simulink library "halin"  (R2021b)
settings: Solver=VariableStepAuto  StartTime=0.0  StopTime=10.0  RelTol=1e-3
undefined symbols (not defined in the file): TRUE
libraries: FVT_lib x177, hcu_lib x55
(part 13 of 17)

== system halin/HAL_IN/CAN1/ESC1/RFPulseCount ==
  RF_PulseCount : Inport
  UnitConverter : DataTypeConversion  OutDataTypeStr=uint8
  VHAL_RFPulseCount_enum : Outport
  wires:
  UnitConverter/1 -> VHAL_RFPulseCount_enum/1
  RF_PulseCount/1 -> UnitConverter/1

== system halin/HAL_IN/CAN1/ESC1/RFPulseCountV ==
  RF_PulseCount_V : Inport
  UnitConverter : DataTypeConversion  OutDataTypeStr=uint8
  VHAL_RFPulseCountV_flg : Outport
  wires:
  UnitConverter/1 -> VHAL_RFPulseCountV_flg/1
  RF_PulseCount_V/1 -> UnitConverter/1

== system halin/HAL_IN/CAN1/ESC1/RFRawWhlSpeed ==
  RF_RawWhlSpeed : Inport
  UnitConverter : DataTypeConversion  OutDataTypeStr=uint16
  convert_in : FVT_lib/hal/convert_in  gain=0.0625  offset=0
  VHAL_RFRawWhlSpeed_kph : Outport
  wires:
  convert_in/1 -> VHAL_RFRawWhlSpeed_kph/1
  UnitConverter/1 -> convert_in/1
  RF_RawWhlSpeed/1 -> UnitConverter/1

== system halin/HAL_IN/CAN1/ESC1/RFRawWhlSpeedV ==
  RF_RawWhlSpeed_V : Inport
  UnitConverter : DataTypeConversion  OutDataTypeStr=uint8
  VHAL_RFRawWhlSpeedV_flg : Outport
  wires:
  UnitConverter/1 -> VHAL_RFRawWhlSpeedV_flg/1
  RF_RawWhlSpeed_V/1 -> UnitConverter/1

== system halin/HAL_IN/CAN1/ESC1/RFWhlRotDir ==
  RF_WhlRotDir : Inport
  UnitConverter : DataTypeConversion  OutDataTypeStr=uint8
  VHAL_RFWhlRotDir_enum : Outport
  wires:
  UnitConverter/1 -> VHAL_RFWhlRotDir_enum/1
  RF_WhlRotDir/1 -> UnitConverter/1

== system halin/HAL_IN/CAN1/ESC1/RRPulseCount ==
  RR_PulseCount : Inport
  UnitConverter : DataTypeConversion  OutDataTypeStr=uint8
  VHAL_RRPulseCount_enum : Outport
  wires:
  UnitConverter/1 -> VHAL_RRPulseCount_enum/1
  RR_PulseCount/1 -> UnitConverter/1

== system halin/HAL_IN/CAN1/ESC1/RRPulseCountV ==
  RR_PulseCount_V : Inport
  UnitConverter : DataTypeConversion  OutDataTypeStr=uint8
  VHAL_RRPulseCountV_flg : Outport
  wires:
  UnitConverter/1 -> VHAL_RRPulseCountV_flg/1
  RR_PulseCount_V/1 -> UnitConverter/1

== system halin/HAL_IN/CAN1/ESC1/RRRawWhlSpeed ==
  RR_RawWhlSpeed : Inport
  UnitConverter : DataTypeConversion  OutDataTypeStr=uint16
  convert_in : FVT_lib/hal/convert_in  gain=0.0625  offset=0
  VHAL_RRRawWhlSpeed_kph : Outport
  wires:
  convert_in/1 -> VHAL_RRRawWhlSpeed_kph/1
  UnitConverter/1 -> convert_in/1
  RR_RawWhlSpeed/1 -> UnitConverter/1

== system halin/HAL_IN/CAN1/ESC1/RRRawWhlSpeedV ==
  RR_RawWhlSpeed_V : Inport
  UnitConverter : DataTypeConversion  OutDataTypeStr=uint8
  VHAL_RRRawWhlSpeedV_flg : Outport
  wires:
  UnitConverter/1 -> VHAL_RRRawWhlSpeedV_flg/1
  RR_RawWhlSpeed_V/1 -> UnitConverter/1

== system halin/HAL_IN/CAN1/ESC1/RRWhlRotDir ==
  RR_WhlRotDir : Inport
  UnitConverter : DataTypeConversion  OutDataTypeStr=uint8
  VHAL_RRWhlRotDir_enum : Outport
  wires:
  UnitConverter/1 -> VHAL_RRWhlRotDir_enum/1
  RR_WhlRotDir/1 -> UnitConverter/1

== system halin/HAL_IN/CAN1/ESC1/RearAxlTrqReqDrv ==
  RearAxlTrqReq_Drv : Inport
  UnitConverter : DataTypeConversion  OutDataTypeStr=uint16
  convert_in : FVT_lib/hal/convert_in  gain=0.5  offset=-5300
  VHAL_RearAxlTrqReqDrv_Nm : Outport
  wires:
  convert_in/1 -> VHAL_RearAxlTrqReqDrv_Nm/1
  UnitConverter/1 -> convert_in/1
  RearAxlTrqReq_Drv/1 -> UnitConverter/1

== system halin/HAL_IN/CAN1/ESC1/RedWnlmpSta ==
  Red_WnlmpSta : Inport
  UnitConverter : DataTypeConversion  OutDataTypeStr=uint8
  VHAL_RedWnlmpSta_flg : Outport
  wires:
  UnitConverter/1 -> VHAL_RedWnlmpSta_flg/1
  Red_WnlmpSta/1 -> UnitConverter/1

== system halin/HAL_IN/CAN1/ESC1/RrPTCSActive ==
  Rr_PTCS_Active : Inport
  UnitConverter : DataTypeConversion  OutDataTypeStr=uint8
  VHAL_RrPTCSActive_flg : Outport
  wires:
  UnitConverter/1 -> VHAL_RrPTCSActive_flg/1
  Rr_PTCS_Active/1 -> UnitConverter/1

== system halin/HAL_IN/CAN1/ESC1/TCSActive ==
  TCS_Active : Inport
  UnitConverter : DataTypeConversion  OutDataTypeStr=uint8
  VHAL_TCSActive_flg : Outport
  wires:
  UnitConverter/1 -> VHAL_TCSActive_flg/1
  TCS_Active/1 -> UnitConverter/1

== system halin/HAL_IN/CAN1/ESC1/TCSFailed ==
  TCS_Failed : Inport
  UnitConverter : DataTypeConversion  OutDataTypeStr=uint8
  VHAL_TCSFailed_flg : Outport
  wires:
  UnitConverter/1 -> VHAL_TCSFailed_flg/1
  TCS_Failed/1 -> UnitConverter/1

== system halin/HAL_IN/CAN1/ESC1/VehSpeed ==
  VehSpeed : Inport
  UnitConverter : DataTypeConversion  OutDataTypeStr=uint16
  convert_in : FVT_lib/hal/convert_in  gain=0.125  offset=0
  VHAL_VehSpeed_kph : Outport
  wires:
  convert_in/1 -> VHAL_VehSpeed_kph/1
  UnitConverter/1 -> convert_in/1
  VehSpeed/1 -> UnitConverter/1

== system halin/HAL_IN/CAN1/ESC5/ACCAvail ==
  ACCAvail : Inport
  UnitConverter : DataTypeConversion  OutDataTypeStr=uint8
  VHAL_ACCAvail_flg : Outport
  wires:
  UnitConverter/1 -> VHAL_ACCAvail_flg/1
  ACCAvail/1 -> UnitConverter/1

== system halin/HAL_IN/CAN1/ESC5/AEBAvail ==
  AEBAvail : Inport
  UnitConverter : DataTypeConversion  OutDataTypeStr=uint8
  VHAL_AEBAvail_flg : Outport
  wires:
  UnitConverter/1 -> VHAL_AEBAvail_flg/1
  AEBAvail/1 -> UnitConverter/1

== system halin/HAL_IN/CAN1/ESC5/ActBrkLampSta ==
  ActBrkLamp_Sta : Inport
  UnitConverter : DataTypeConversion  OutDataTypeStr=uint8
  VHAL_ActBrkLampSta_flg : Outport
  wires:
  UnitConverter/1 -> VHAL_ActBrkLampSta_flg/1
  ActBrkLamp_Sta/1 -> UnitConverter/1

== system halin/HAL_IN/CAN1/ESC5/BrkDiscTempSta ==
  BrkDiscTempSta : Inport
  UnitConverter : DataTypeConversion  OutDataTypeStr=uint8
  VHAL_BrkDiscTempSta_flg : Outport
  wires:
  UnitConverter/1 -> VHAL_BrkDiscTempSta_flg/1
  BrkDiscTempSta/1 -> UnitConverter/1

== system halin/HAL_IN/CAN1/ESC5/BrkPedalPos ==
  BrkPedalPos : Inport
  UnitConverter : DataTypeConversion  OutDataTypeStr=uint8
  convert_in : FVT_lib/hal/convert_in  gain=0.4  offset=0
  VHAL_BrkPedalPos_pct : Outport
  wires:
  convert_in/1 -> VHAL_BrkPedalPos_pct/1
  UnitConverter/1 -> convert_in/1
  BrkPedalPos/1 -> UnitConverter/1

== system halin/HAL_IN/CAN1/ESC5/BrkPedalPosSta ==
  BrkPedalPos_Sta : Inport
  UnitConverter : DataTypeConversion  OutDataTypeStr=uint8
  VHAL_BrkPedalPosSta_flg : Outport
  wires:
  UnitConverter/1 -> VHAL_BrkPedalPosSta_flg/1
  BrkPedalPos_Sta/1 -> UnitConverter/1

== system halin/HAL_IN/CAN1/ESC5/BrkSwSta ==
  BrkSw_Sta : Inport
  UnitConverter : DataTypeConversion  OutDataTypeStr=uint8
  VHAL_BrkSwSta_flg : Outport
  wires:
  UnitConverter/1 -> VHAL_BrkSwSta_flg/1
  BrkSw_Sta/1 -> UnitConverter/1

== system halin/HAL_IN/CAN1/ESC5/BrkSwV ==
  BrkSw_V : Inport
  UnitConverter : DataTypeConversion  OutDataTypeStr=uint8
  VHAL_BrkSwV_flg : Outport
  wires:
  UnitConverter/1 -> VHAL_BrkSwV_flg/1
  BrkSw_V/1 -> UnitConverter/1

== system halin/HAL_IN/CAN1/ESC5/ESC5CS ==
  ESC5_CS : Inport
  UnitConverter : DataTypeConversion  OutDataTypeStr=uint8
  VHAL_ESC5CS_enum : Outport
  wires:
  UnitConverter/1 -> VHAL_ESC5CS_enum/1
  ESC5_CS/1 -> UnitConverter/1

== system halin/HAL_IN/CAN1/ESC5/ESC5RC ==
  ESC5_RC : Inport
  UnitConverter : DataTypeConversion  OutDataTypeStr=uint8
  VHAL_ESC5RC_enum : Outport
  wires:
  UnitConverter/1 -> VHAL_ESC5RC_enum/1
  ESC5_RC/1 -> UnitConverter/1

== system halin/HAL_IN/CAN1/ESC5/ESCADASSta ==
  ESC_ADAS_Sta : Inport
  UnitConverter : DataTypeConversion  OutDataTypeStr=uint8
  VHAL_ESCADASSta_enum : Outport
  wires:
  UnitConverter/1 -> VHAL_ESCADASSta_enum/1
  ESC_ADAS_Sta/1 -> UnitConverter/1

== system halin/HAL_IN/CAN1/ESC5/ESCAPSSta ==
  ESC_APS_Sta : Inport
  UnitConverter : DataTypeConversion  OutDataTypeStr=uint8
  VHAL_ESCAPSSta_enum : Outport
  wires:
  UnitConverter/1 -> VHAL_ESCAPSSta_enum/1
  ESC_APS_Sta/1 -> UnitConverter/1

== system halin/HAL_IN/CAN1/ESC5/ESCStandstill ==
  ESC_Standstill : Inport
  UnitConverter : DataTypeConversion  OutDataTypeStr=uint8
  VHAL_ESCStandstill_flg : Outport
  wires:
  UnitConverter/1 -> VHAL_ESCStandstill_flg/1
  ESC_Standstill/1 -> UnitConverter/1

== system halin/HAL_IN/CAN1/ESC5/FrRBCActive ==
  Fr_RBC_Active : Inport
  UnitConverter : DataTypeConversion  OutDataTypeStr=uint8
  VHAL_FrRBCActive_flg : Outport
  wires:
  UnitConverter/1 -> VHAL_FrRBCActive_flg/1
  Fr_RBC_Active/1 -> UnitConverter/1

== system halin/HAL_IN/CAN1/ESC5/FrntAxlTrqReqBrk ==
  FrntAxlTrqReq_Brk : Inport
  UnitConverter : DataTypeConversion  OutDataTypeStr=uint16
  convert_in : FVT_lib/hal/convert_in  gain=0.5  offset=-5300
  VHAL_FrntAxlTrqReqBrk_Nm : Outport
  wires:
  convert_in/1 -> VHAL_FrntAxlTrqReqBrk_Nm/1
  UnitConverter/1 -> convert_in/1
  FrntAxlTrqReq_Brk/1 -> UnitConverter/1

== system halin/HAL_IN/CAN1/ESC5/LatAccel ==
  LatAccel : Inport
  UnitConverter : DataTypeConversion  OutDataTypeStr=uint8
  convert_in : FVT_lib/hal/convert_in  gain=0.01  offset=-1.27
  VHAL_LatAccel_Gps : Outport
  wires:
  convert_in/1 -> VHAL_LatAccel_Gps/1
  UnitConverter/1 -> convert_in/1
  LatAccel/1 -> UnitConverter/1

== system halin/HAL_IN/CAN1/ESC5/LatAccelV ==
  LatAccel_V : Inport
  UnitConverter : DataTypeConversion  OutDataTypeStr=uint8
  VHAL_LatAccelV_flg : Outport
  wires:
  UnitConverter/1 -> VHAL_LatAccelV_flg/1
  LatAccel_V/1 -> UnitConverter/1

== system halin/HAL_IN/CAN1/ESC5/LongAccel ==
  LongAccel : Inport
  UnitConverter : DataTypeConversion  OutDataTypeStr=uint8
  convert_in : FVT_lib/hal/convert_in  gain=0.01  offset=-1.27
  VHAL_LongAccel_Gps : Outport
  wires:
  convert_in/1 -> VHAL_LongAccel_Gps/1
  UnitConverter/1 -> convert_in/1
  LongAccel/1 -> UnitConverter/1

== system halin/HAL_IN/CAN1/ESC5/LongAccelV ==
  LongAccel_V : Inport
  UnitConverter : DataTypeConversion  OutDataTypeStr=uint8
  VHAL_LongAccelV_flg : Outport
  wires:
  UnitConverter/1 -> VHAL_LongAccelV_flg/1
  LongAccel_V/1 -> UnitConverter/1

== system halin/HAL_IN/CAN1/ESC5/MCPressure ==
  MCPressure : Inport
  UnitConverter : DataTypeConversion  OutDataTypeStr=uint16
  convert_in : FVT_lib/hal/convert_in  gain=0.1  offset=-9.7
  VHAL_MCPressure_bar : Outport
  wires:
  convert_in/1 -> VHAL_MCPressure_bar/1
  UnitConverter/1 -> convert_in/1
  MCPressure/1 -> UnitConverter/1

== system halin/HAL_IN/CAN1/ESC5/MCPressureV ==
  MCPressure_V : Inport
  UnitConverter : DataTypeConversion  OutDataTypeStr=uint8
  VHAL_MCPressureV_flg : Outport
  wires:
  UnitConverter/1 -> VHAL_MCPressureV_flg/1
  MCPressure_V/1 -> UnitConverter/1

== system halin/HAL_IN/CAN1/ESC5/MeterIndVehSpeed ==
  Meter_Ind_VehSpeed : Inport
  UnitConverter : DataTypeConversion  OutDataTypeStr=uint16
  convert_in : FVT_lib/hal/convert_in  gain=0.125  offset=0
  VHAL_MeterIndVehSpeed_kph : Outport
  wires:
  convert_in/1 -> VHAL_MeterIndVehSpeed_kph/1
  UnitConverter/1 -> convert_in/1
  Meter_Ind_VehSpeed/1 -> UnitConverter/1

== system halin/HAL_IN/CAN1/ESC5/RDCActive ==
  RDC_Active : Inport
  UnitConverter : DataTypeConversion  OutDataTypeStr=uint8
  VHAL_RDCActive_enum : Outport
  wires:
  UnitConverter/1 -> VHAL_RDCActive_enum/1
  RDC_Active/1 -> UnitConverter/1

== system halin/HAL_IN/CAN1/ESC5/RearAxlTrqReqBrk ==
  RearAxlTrqReq_Brk : Inport
  UnitConverter : DataTypeConversion  OutDataTypeStr=uint16
  convert_in : FVT_lib/hal/convert_in  gain=0.5  offset=-5300
  VHAL_RearAxlTrqReqBrk_Nm : Outport
  wires:
  convert_in/1 -> VHAL_RearAxlTrqReqBrk_Nm/1
  UnitConverter/1 -> convert_in/1
  RearAxlTrqReq_Brk/1 -> UnitConverter/1

== system halin/HAL_IN/CAN1/ESC5/RrRBCActive ==
  Rr_RBC_Active : Inport
  UnitConverter : DataTypeConversion  OutDataTypeStr=uint8
  VHAL_RrRBCActive_flg : Outport
  wires:
  UnitConverter/1 -> VHAL_RrRBCActive_flg/1
  Rr_RBC_Active/1 -> UnitConverter/1

== system halin/HAL_IN/CAN1/ESC5/YawRate ==
  YawRate : Inport
  UnitConverter : DataTypeConversion  OutDataTypeStr=uint16
  convert_in : FVT_lib/hal/convert_in  gain=0.1  offset=-100
  VHAL_YawRate_degps : Outport
  wires:
  convert_in/1 -> VHAL_YawRate_degps/1
  UnitConverter/1 -> convert_in/1
  YawRate/1 -> UnitConverter/1

== system halin/HAL_IN/CAN1/ESC5/YawRateV ==
  YawRate_V : Inport
  UnitConverter : DataTypeConversion  OutDataTypeStr=uint8
  VHAL_YawRateV_flg : Outport
  wires:
  UnitConverter/1 -> VHAL_YawRateV_flg/1
  YawRate_V/1 -> UnitConverter/1

== system halin/HAL_IN/CAN1/eBST1/LowBrakeFluidSta ==
  LowBrakeFluid_Sta : Inport
  UnitConverter : DataTypeConversion  OutDataTypeStr=uint8
  VHAL_LowBrakeFluidSta_flg : Outport
  wires:
  UnitConverter/1 -> VHAL_LowBrakeFluidSta_flg/1
  LowBrakeFluid_Sta/1 -> UnitConverter/1

== system halin/HAL_IN/CAN1/eBST1/eBSTAmberWnlmpSta ==
  eBST_AmberWnlmpSta : Inport
  UnitConverter : DataTypeConversion  OutDataTypeStr=uint8
  VHAL_eBSTAmberWnlmpSta_flg : Outport
  wires:
  UnitConverter/1 -> VHAL_eBSTAmberWnlmpSta_flg/1
  eBST_AmberWnlmpSta/1 -> UnitConverter/1

== system halin/HAL_IN/CAN1/eBST1/eBSTBeepReq ==
  eBST_BeepReq : Inport
  UnitConverter : DataTypeConversion  OutDataTypeStr=uint8
  VHAL_eBSTBeepReq_flg : Outport
  wires:
  UnitConverter/1 -> VHAL_eBSTBeepReq_flg/1
  eBST_BeepReq/1 -> UnitConverter/1

== system halin/HAL_IN/CAN1/eBST1/eBSTRedWnlmpSta ==
  eBST_RedWnlmpSta : Inport
  UnitConverter : DataTypeConversion  OutDataTypeStr=uint8
  VHAL_eBSTRedWnlmpSta_flg : Outport
  wires:
  UnitConverter/1 -> VHAL_eBSTRedWnlmpSta_flg/1
  eBST_RedWnlmpSta/1 -> UnitConverter/1

== system halin/HAL_IN/CAN2/HMI1/HMIACAirIntMCmd ==
  HMI_ACAirIntM_Cmd : Inport
  UnitConverter : DataTypeConversion  OutDataTypeStr=uint8
  VHAL_HMIACAirIntMCmd_flg : Outport
  wires:
  UnitConverter/1 -> VHAL_HMIACAirIntMCmd_flg/1
  HMI_ACAirIntM_Cmd/1 -> UnitConverter/1

== system halin/HAL_IN/CAN2/HMI1/HMIACAirIntPCmd ==
  HMI_ACAirIntP_Cmd : Inport
  UnitConverter : DataTypeConversion  OutDataTypeStr=uint8
  VHAL_HMIACAirIntPCmd_flg : Outport
  wires:
  UnitConverter/1 -> VHAL_HMIACAirIntPCmd_flg/1
  HMI_ACAirIntP_Cmd/1 -> UnitConverter/1

== system halin/HAL_IN/CAN2/HMI1/HMIACAutoBtnCmd ==
  HMI_ACAutoBtn_Cmd : Inport
  UnitConverter : DataTypeConversion  OutDataTypeStr=uint8
  VHAL_HMIACAutoBtnCmd_flg : Outport
  wires:
  UnitConverter/1 -> VHAL_HMIACAutoBtnCmd_flg/1
  HMI_ACAutoBtn_Cmd/1 -> UnitConverter/1

== system halin/HAL_IN/CAN2/HMI1/HMIACBtnCmd ==
  HMI_ACBtn_Cmd : Inport
  UnitConverter : DataTypeConversion  OutDataTypeStr=uint8
  VHAL_HMIACBtnCmd_flg : Outport
  wires:
  UnitConverter/1 -> VHAL_HMIACBtnCmd_flg/1
  HMI_ACBtn_Cmd/1 -> UnitConverter/1

== system halin/HAL_IN/CAN2/HMI1/HMIACFrDefogBtnCmd ==
  HMI_ACFrDefogBtn_Cmd : Inport
  UnitConverter : DataTypeConversion  OutDataTypeStr=uint8
  VHAL_HMIACFrDefogBtnCmd_flg : Outport
  wires:
  UnitConverter/1 -> VHAL_HMIACFrDefogBtnCmd_flg/1
  HMI_ACFrDefogBtn_Cmd/1 -> UnitConverter/1

== system halin/HAL_IN/CAN2/HMI1/HMIACRecycleBtnCmd ==
  HMI_ACRecycleBtn_Cmd : Inport
  UnitConverter : DataTypeConversion  OutDataTypeStr=uint8
  VHAL_HMIACRecycleBtnCmd_flg : Outport
  wires:
  UnitConverter/1 -> VHAL_HMIACRecycleBtnCmd_flg/1
  HMI_ACRecycleBtn_Cmd/1 -> UnitConverter/1

== system halin/HAL_IN/CAN2/HMI1/HMIACWindDirMCmd ==
  HMI_ACWindDirM_Cmd : Inport
  UnitConverter : DataTypeConversion  OutDataTypeStr=uint8
  VHAL_HMIACWindDirMCmd_flg : Outport
  wires:
  UnitConverter/1 -> VHAL_HMIACWindDirMCmd_flg/1
  HMI_ACWindDirM_Cmd/1 -> UnitConverter/1

== system halin/HAL_IN/CAN2/HMI1/HMIACWindDirPCmd ==
  HMI_ACWindDirP_Cmd : Inport
  UnitConverter : DataTypeConversion  OutDataTypeStr=uint8
  VHAL_HMIACWindDirPCmd_flg : Outport
  wires:
  UnitConverter/1 -> VHAL_HMIACWindDirPCmd_flg/1
  HMI_ACWindDirP_Cmd/1 -> UnitConverter/1

== system halin/HAL_IN/CAN2/HMI1/HMIZ1SetTMCmd ==
  HMI_Z1SetTM_Cmd : Inport
  UnitConverter : DataTypeConversion  OutDataTypeStr=uint8
  VHAL_HMIZ1SetTMCmd_flg : Outport
  wires:
  UnitConverter/1 -> VHAL_HMIZ1SetTMCmd_flg/1
  HMI_Z1SetTM_Cmd/1 -> UnitConverter/1

== system halin/HAL_IN/CAN2/HMI1/HMIZ1SetTPCmd ==
  HMI_Z1SetTP_Cmd : Inport
  UnitConverter : DataTypeConversion  OutDataTypeStr=uint8
  VHAL_HMIZ1SetTPCmd_flg : Outport
  wires:
  UnitConverter/1 -> VHAL_HMIZ1SetTPCmd_flg/1
  HMI_Z1SetTP_Cmd/1 -> UnitConverter/1

== system halin/HAL_IN/CAN2/HMI1/HMIZ2SetTMCmd ==
  HMI_Z2SetTM_Cmd : Inport
  UnitConverter : DataTypeConversion  OutDataTypeStr=uint8
  VHAL_HMIZ2SetTMCmd_flg : Outport
  wires:
  UnitConverter/1 -> VHAL_HMIZ2SetTMCmd_flg/1
  HMI_Z2SetTM_Cmd/1 -> UnitConverter/1

== system halin/HAL_IN/CAN2/HMI1/HMIZ2SetTPCmd ==
  HMI_Z2SetTP_Cmd : Inport
  UnitConverter : DataTypeConversion  OutDataTypeStr=uint8
  VHAL_HMIZ2SetTPCmd_flg : Outport
  wires:
  UnitConverter/1 -> VHAL_HMIZ2SetTPCmd_flg/1
  HMI_Z2SetTP_Cmd/1 -> UnitConverter/1

== system halin/HAL_IN/CAN2/IVI1/AmbLighLowBatAlertSW ==
  AmbLigh_LowBatAlert_SW : Inport
  UnitConverter : DataTypeConversion  OutDataTypeStr=uint8
  VHAL_AmbLighLowBatAlertSW_flg : Outport
  wires:
  UnitConverter/1 -> VHAL_AmbLighLowBatAlertSW_flg/1
  AmbLigh_LowBatAlert_SW/1 -> UnitConverter/1

== system halin/HAL_IN/CAN2/IVI1/AmbLighSafetyAlertSW ==
  AmbLigh_SafetyAlert_SW : Inport
  UnitConverter : DataTypeConversion  OutDataTypeStr=uint8
  VHAL_AmbLighSafetyAlertSW_flg : Outport
  wires:
  UnitConverter/1 -> VHAL_AmbLighSafetyAlertSW_flg/1
  AmbLigh_SafetyAlert_SW/1 -> UnitConverter/1

== system halin/HAL_IN/CAN2/IVI1/AmbLightBrightnessSet ==
  AmbLightBrightnessSet : Inport
  UnitConverter : DataTypeConversion  OutDataTypeStr=uint8
  VHAL_AmbLightBrightnessSet_enum : Outport
  wires:
  UnitConverter/1 -> VHAL_AmbLightBrightnessSet_enum/1
  AmbLightBrightnessSet/1 -> UnitConverter/1

== system halin/HAL_IN/CAN2/IVI1/AmbLightColorSet ==
  AmbLightColorSet : Inport
  UnitConverter : DataTypeConversion  OutDataTypeStr=uint8
  VHAL_AmbLightColorSet_enum : Outport
  wires:
  UnitConverter/1 -> VHAL_AmbLightColorSet_enum/1
  AmbLightColorSet/1 -> UnitConverter/1

== system halin/HAL_IN/CAN2/IVI1/AmbLightDimInDarkSW ==
  AmbLight_DimInDark_SW : Inport
  UnitConverter : DataTypeConversion  OutDataTypeStr=uint8
  VHAL_AmbLightDimInDarkSW_flg : Outport
  wires:
  UnitConverter/1 -> VHAL_AmbLightDimInDarkSW_flg/1
  AmbLight_DimInDark_SW/1 -> UnitConverter/1

== system halin/HAL_IN/CAN2/IVI1/AmbLightSW ==
  AmbLight_SW : Inport
  UnitConverter : DataTypeConversion  OutDataTypeStr=uint8
  VHAL_AmbLightSW_flg : Outport
  wires:
  UnitConverter/1 -> VHAL_AmbLightSW_flg/1
  AmbLight_SW/1 -> UnitConverter/1

== system halin/HAL_IN/CAN2/IVI1/AmbLightWlcmLightSW ==
  AmbLight_WlcmLight_SW : Inport
  UnitConverter : DataTypeConversion  OutDataTypeStr=uint8
  VHAL_AmbLightWlcmLightSW_flg : Outport
  wires:
  UnitConverter/1 -> VHAL_AmbLightWlcmLightSW_flg/1
  AmbLight_WlcmLight_SW/1 -> UnitConverter/1

== system halin/HAL_IN/CAN2/IVI1/FCPFrEvtBtnACMaxReq ==
  FCP_FrEvt_BtnACMaxReq : Inport
  UnitConverter : DataTypeConversion  OutDataTypeStr=uint8
  VHAL_FCPFrEvtBtnACMaxReq_flg : Outport
  wires:
  UnitConverter/1 -> VHAL_FCPFrEvtBtnACMaxReq_flg/1
  FCP_FrEvt_BtnACMaxReq/1 -> UnitConverter/1

== system halin/HAL_IN/CAN2/IVI1/FCPFrEvtBtnACReq ==
  FCP_FrEvt_BtnACReq : Inport
  UnitConverter : DataTypeConversion  OutDataTypeStr=uint8
  VHAL_FCPFrEvtBtnACReq_flg : Outport
  wires:
  UnitConverter/1 -> VHAL_FCPFrEvtBtnACReq_flg/1
  FCP_FrEvt_BtnACReq/1 -> UnitConverter/1

== system halin/HAL_IN/CAN2/IVI1/FCPFrEvtBtnAutoReq ==
  FCP_FrEvt_BtnAutoReq : Inport
  UnitConverter : DataTypeConversion  OutDataTypeStr=uint8
  VHAL_FCPFrEvtBtnAutoReq_flg : Outport
  wires:
  UnitConverter/1 -> VHAL_FCPFrEvtBtnAutoReq_flg/1
  FCP_FrEvt_BtnAutoReq/1 -> UnitConverter/1

== system halin/HAL_IN/CAN2/IVI1/FCPFrEvtBtnSyncReq ==
  FCP_FrEvt_BtnSyncReq : Inport
  UnitConverter : DataTypeConversion  OutDataTypeStr=uint8
  VHAL_FCPFrEvtBtnSyncReq_flg : Outport
  wires:
  UnitConverter/1 -> VHAL_FCPFrEvtBtnSyncReq_flg/1
  FCP_FrEvt_BtnSyncReq/1 -> UnitConverter/1

== system halin/HAL_IN/CAN2/IVI1/IVICreateAccReqSta ==
  IVI_CreateAccReq_Sta : Inport
  UnitConverter : DataTypeConversion  OutDataTypeStr=uint8
  VHAL_IVICreateAccReqSta_enum : Outport
  wires:
  UnitConverter/1 -> VHAL_IVICreateAccReqSta_enum/1
  IVI_CreateAccReq_Sta/1 -> UnitConverter/1

== system halin/HAL_IN/CAN2/IVI1/IVIDelAccReqSta ==
  IVI_DelAccReq_Sta : Inport
  UnitConverter : DataTypeConversion  OutDataTypeStr=uint8
  VHAL_IVIDelAccReqSta_enum : Outport
  wires:
  UnitConverter/1 -> VHAL_IVIDelAccReqSta_enum/1
  IVI_DelAccReq_Sta/1 -> UnitConverter/1

== system halin/HAL_IN/CAN2/IVI1/IVILinkAccReqSta ==
  IVI_LinkAccReq_Sta : Inport
  UnitConverter : DataTypeConversion  OutDataTypeStr=uint8
  VHAL_IVILinkAccReqSta_flg : Outport
  wires:
  UnitConverter/1 -> VHAL_IVILinkAccReqSta_flg/1
  IVI_LinkAccReq_Sta/1 -> UnitConverter/1

== system halin/HAL_IN/CAN2/IVI1/IVILinkAccSta ==
  IVI_LinkAcc_Sta : Inport
  UnitConverter : DataTypeConversion  OutDataTypeStr=uint8
  VHAL_IVILinkAccSta_enum : Outport
  wires:
  UnitConverter/1 -> VHAL_IVILinkAccSta_enum/1
  IVI_LinkAcc_Sta/1 -> UnitConverter/1

== system halin/HAL_IN/CAN2/IVI1/IVILinkKeySta ==
  IVI_LinkKey_Sta : Inport
  UnitConverter : DataTypeConversion  OutDataTypeStr=uint8
  VHAL_IVILinkKeySta_enum : Outport
  wires:
  UnitConverter/1 -> VHAL_IVILinkKeySta_enum/1
  IVI_LinkKey_Sta/1 -> UnitConverter/1

== system halin/HAL_IN/CAN2/IVI1/IVILocatedSTA ==
  IVI_Located_STA : Inport
  UnitConverter : DataTypeConversion  OutDataTypeStr=uint8
  VHAL_IVILocatedSTA_enum : Outport
  wires:
  UnitConverter/1 -> VHAL_IVILocatedSTA_enum/1
  IVI_Located_STA/1 -> UnitConverter/1

== system halin/HAL_IN/CAN2/IVI1/IVILockSoundSWSta ==
  IVI_Lock_SoundSW_Sta : Inport
  UnitConverter : DataTypeConversion  OutDataTypeStr=uint8
  VHAL_IVILockSoundSWSta_flg : Outport
  wires:
  UnitConverter/1 -> VHAL_IVILockSoundSWSta_flg/1
  IVI_Lock_SoundSW_Sta/1 -> UnitConverter/1

== system halin/HAL_IN/CAN2/IVI1/IVITimeCheck ==
  IVI_Time_Check : Inport
  UnitConverter : DataTypeConversion  OutDataTypeStr=uint8
  VHAL_IVITimeCheck_enum : Outport
  wires:
  UnitConverter/1 -> VHAL_IVITimeCheck_enum/1
  IVI_Time_Check/1 -> UnitConverter/1

== system halin/HAL_IN/CAN2/IVI1/IVITimeDay ==
  IVI_Time_Day : Inport
  UnitConverter : DataTypeConversion  OutDataTypeStr=uint8
  VHAL_IVITimeDay_DAY : Outport
  wires:
  UnitConverter/1 -> VHAL_IVITimeDay_DAY/1
  IVI_Time_Day/1 -> UnitConverter/1

== system halin/HAL_IN/CAN2/IVI1/IVITimeHour ==
  IVI_Time_Hour : Inport
  UnitConverter : DataTypeConversion  OutDataTypeStr=uint8
  VHAL_IVITimeHour_hr : Outport
  wires:
  UnitConverter/1 -> VHAL_IVITimeHour_hr/1
  IVI_Time_Hour/1 -> UnitConverter/1

== system halin/HAL_IN/CAN2/IVI1/IVITimeMinute ==
  IVI_Time_Minute : Inport
  UnitConverter : DataTypeConversion  OutDataTypeStr=uint8
  VHAL_IVITimeMinute_min : Outport
  wires:
  UnitConverter/1 -> VHAL_IVITimeMinute_min/1
  IVI_Time_Minute/1 -> UnitConverter/1

== system halin/HAL_IN/CAN2/IVI1/IVITimeMonth ==
  IVI_Time_Month : Inport
  UnitConverter : DataTypeConversion  OutDataTypeStr=uint8
  VHAL_IVITimeMonth_MONTH : Outport
  wires:
  UnitConverter/1 -> VHAL_IVITimeMonth_MONTH/1
  IVI_Time_Month/1 -> UnitConverter/1

== system halin/HAL_IN/CAN2/IVI1/IVITimeSecond ==
  IVI_Time_Second : Inport
  UnitConverter : DataTypeConversion  OutDataTypeStr=uint8
  VHAL_IVITimeSecond_s : Outport
  wires:
  UnitConverter/1 -> VHAL_IVITimeSecond_s/1
  IVI_Time_Second/1 -> UnitConverter/1

== system halin/HAL_IN/CAN2/IVI1/IVITimeYear ==
  IVI_Time_Year : Inport
  UnitConverter : DataTypeConversion  OutDataTypeStr=uint8
  convert_in : FVT_lib/hal/convert_in  gain=1  offset=2000
  VHAL_IVITimeYear_YEAR : Outport
  wires:
  convert_in/1 -> VHAL_IVITimeYear_YEAR/1
  UnitConverter/1 -> convert_in/1
  IVI_Time_Year/1 -> UnitConverter/1

== system halin/HAL_IN/CAN2/IVI1/LINKtoDrive ==
  LINKtoDrive : Inport
  UnitConverter : DataTypeConversion  OutDataTypeStr=uint8
  VHAL_LINKtoDrive_flg : Outport
  wires:
  UnitConverter/1 -> VHAL_LINKtoDrive_flg/1
  LINKtoDrive/1 -> UnitConverter/1

== system halin/HAL_IN/CAN2/IVI1/OpenDrOpenWdoSW ==
  OpenDrOpenWdo_SW : Inport
  UnitConverter : DataTypeConversion  OutDataTypeStr=uint8
  VHAL_OpenDrOpenWdoSW_flg : Outport
  wires:
  UnitConverter/1 -> VHAL_OpenDrOpenWdoSW_flg/1
  OpenDrOpenWdo_SW/1 -> UnitConverter/1

== system halin/HAL_IN/CAN2/IVI1/PWCONTINUEUSE ==
  PW_CONTINUE_USE : Inport
  UnitConverter : DataTypeConversion  OutDataTypeStr=uint8
  VHAL_PWCONTINUEUSE_flg : Outport
  wires:
  UnitConverter/1 -> VHAL_PWCONTINUEUSE_flg/1
  PW_CONTINUE_USE/1 -> UnitConverter/1

== system halin/HAL_IN/CAN2/IVI1/SmartEcoModeSW ==
  SmartEco_Mode_SW : Inport
  UnitConverter : DataTypeConversion  OutDataTypeStr=uint8
  VHAL_SmartEcoModeSW_flg : Outport
  wires:
  UnitConverter/1 -> VHAL_SmartEcoModeSW_flg/1
  SmartEco_Mode_SW/1 -> UnitConverter/1

== system halin/HAL_IN/CAN2/IVI1/UserSet ==
  UserSet : Inport
  UnitConverter : DataTypeConversion  OutDataTypeStr=uint8
  VHAL_UserSet_enum : Outport
  wires:
  UnitConverter/1 -> VHAL_UserSet_enum/1
  UserSet/1 -> UnitConverter/1

== system halin/HAL_IN/CAN2/IVI2/ACChgCurSet ==
  AC_Chg_Cur_Set : Inport
  UnitConverter : DataTypeConversion  OutDataTypeStr=uint8
  convert_in : FVT_lib/hal/convert_in  gain=1  offset=5
  VHAL_ACChgCurSet_A : Outport
  wires:
  convert_in/1 -> VHAL_ACChgCurSet_A/1
  UnitConverter/1 -> convert_in/1
  AC_Chg_Cur_Set/1 -> UnitConverter/1

== system halin/HAL_IN/CAN2/IVI2/AVMErrSTA ==
  AVM_Err_STA : Inport
  UnitConverter : DataTypeConversion  OutDataTypeStr=uint8
  VHAL_AVMErrSTA_flg : Outport
  wires:
  UnitConverter/1 -> VHAL_AVMErrSTA_flg/1
  AVM_Err_STA/1 -> UnitConverter/1

== system halin/HAL_IN/CAN2/IVI2/AVMOFFRecButt ==
  AVM_OFF_Rec_Butt : Inport
  UnitConverter : DataTypeConversion  OutDataTypeStr=uint8
  VHAL_AVMOFFRecButt_flg : Outport
  wires:
  UnitConverter/1 -> VHAL_AVMOFFRecButt_flg/1
  AVM_OFF_Rec_Butt/1 -> UnitConverter/1

== system halin/HAL_IN/CAN2/IVI2/AVMParkingmode ==
  AVM_Parking_mode : Inport
  UnitConverter : DataTypeConversion  OutDataTypeStr=uint8
  VHAL_AVMParkingmode_enum : Outport
  wires:
  UnitConverter/1 -> VHAL_AVMParkingmode_enum/1
  AVM_Parking_mode/1 -> UnitConverter/1

== system halin/HAL_IN/CAN2/IVI2/AVMparkingcancel ==
  AVM_parking_cancel : Inport
  UnitConverter : DataTypeConversion  OutDataTypeStr=uint8
  VHAL_AVMparkingcancel_enum : Outport
  wires:
  UnitConverter/1 -> VHAL_AVMparkingcancel_enum/1
  AVM_parking_cancel/1 -> UnitConverter/1

== system halin/HAL_IN/CAN2/IVI2/AVMparkingexcute ==
  AVM_parking_excute : Inport
  UnitConverter : DataTypeConversion  OutDataTypeStr=uint8
  VHAL_AVMparkingexcute_enum : Outport
  wires:
  UnitConverter/1 -> VHAL_AVMparkingexcute_enum/1
  AVM_parking_excute/1 -> UnitConverter/1

== system halin/HAL_IN/CAN2/IVI2/ApproachUnlockSW ==
  Approach_Unlock_SW : Inport
  UnitConverter : DataTypeConversion  OutDataTypeStr=uint8
  VHAL_ApproachUnlockSW_flg : Outport
  wires:
  UnitConverter/1 -> VHAL_ApproachUnlockSW_flg/1
  Approach_Unlock_SW/1 -> UnitConverter/1

== system halin/HAL_IN/CAN2/IVI2/CAASSw ==
  CAAS_Sw : Inport
  UnitConverter : DataTypeConversion  OutDataTypeStr=uint8
  VHAL_CAASSw_enum : Outport
  wires:
  UnitConverter/1 -> VHAL_CAASSw_enum/1
  CAAS_Sw/1 -> UnitConverter/1

== system halin/HAL_IN/CAN2/IVI2/CDLLockButt ==
  CDL_Lock_Butt : Inport
  UnitConverter : DataTypeConversion  OutDataTypeStr=uint8
  VHAL_CDLLockButt_flg : Outport
  wires:
  UnitConverter/1 -> VHAL_CDLLockButt_flg/1
  CDL_Lock_Butt/1 -> UnitConverter/1

== system halin/HAL_IN/CAN2/IVI2/CDLUnlockButt ==
  CDL_Unlock_Butt : Inport
  UnitConverter : DataTypeConversion  OutDataTypeStr=uint8
  VHAL_CDLUnlockButt_flg : Outport
  wires:
  UnitConverter/1 -> VHAL_CDLUnlockButt_flg/1
  CDL_Unlock_Butt/1 -> UnitConverter/1

== system halin/HAL_IN/CAN2/IVI2/DSEATantiset ==
  DSEAT_anti_set : Inport
  UnitConverter : DataTypeConversion  OutDataTypeStr=uint8
  VHAL_DSEATantiset_flg : Outport
  wires:
  UnitConverter/1 -> VHAL_DSEATantiset_flg/1
  DSEAT_anti_set/1 -> UnitConverter/1

== system halin/HAL_IN/CAN2/IVI2/DSEATentryfunset ==
  DSEAT_entryfun_set : Inport
  UnitConverter : DataTypeConversion  OutDataTypeStr=uint8
  VHAL_DSEATentryfunset_flg : Outport
  wires:
  UnitConverter/1 -> VHAL_DSEATentryfunset_flg/1
  DSEAT_entryfun_set/1 -> UnitConverter/1

== system halin/HAL_IN/CAN2/IVI2/DSEATventreq ==
  DSEAT_vent_req : Inport
  UnitConverter : DataTypeConversion  OutDataTypeStr=uint8
  VHAL_DSEATventreq_enum : Outport
  wires:
  UnitConverter/1 -> VHAL_DSEATventreq_enum/1
  DSEAT_vent_req/1 -> UnitConverter/1

== system halin/HAL_IN/CAN2/IVI2/Distanceunit ==
  Distance_unit : Inport
  UnitConverter : DataTypeConversion  OutDataTypeStr=uint8
  VHAL_Distanceunit_flg : Outport
  wires:
  UnitConverter/1 -> VHAL_Distanceunit_flg/1
  Distance_unit/1 -> UnitConverter/1

== system halin/HAL_IN/CAN2/IVI2/ESCSWCmd ==
  ESC_SW_Cmd : Inport
  UnitConverter : DataTypeConversion  OutDataTypeStr=uint8
  VHAL_ESCSWCmd_enum : Outport
  wires:
  UnitConverter/1 -> VHAL_ESCSWCmd_enum/1
  ESC_SW_Cmd/1 -> UnitConverter/1

== system halin/HAL_IN/CAN2/IVI2/FSOffSw ==
  FS_Off_Sw : Inport
  UnitConverter : DataTypeConversion  OutDataTypeStr=uint8
  VHAL_FSOffSw_enum : Outport
  wires:
  UnitConverter/1 -> VHAL_FSOffSw_enum/1
  FS_Off_Sw/1 -> UnitConverter/1

== system halin/HAL_IN/CAN2/IVI2/FollowMeSW ==
  FollowMeSW : Inport
  UnitConverter : DataTypeConversion  OutDataTypeStr=uint8
  VHAL_FollowMeSW_flg : Outport
  wires:
  UnitConverter/1 -> VHAL_FollowMeSW_flg/1
  FollowMeSW/1 -> UnitConverter/1

== system halin/HAL_IN/CAN2/IVI2/GPSLAT ==
  GPS_LAT : Inport
  UnitConverter : DataTypeConversion  OutDataTypeStr=uint32
  VHAL_GPSLAT_s : Outport
  wires:
  UnitConverter/1 -> VHAL_GPSLAT_s/1
  GPS_LAT/1 -> UnitConverter/1

== system halin/HAL_IN/CAN2/IVI2/GPSLONG ==
  GPS_LONG : Inport
  UnitConverter : DataTypeConversion  OutDataTypeStr=uint32
  VHAL_GPSLONG_enum : Outport
  wires:
  UnitConverter/1 -> VHAL_GPSLONG_enum/1
  GPS_LONG/1 -> UnitConverter/1

== system halin/HAL_IN/CAN2/IVI2/HeadLampSW ==
  HeadLampSW : Inport
  UnitConverter : DataTypeConversion  OutDataTypeStr=uint8
  VHAL_HeadLampSW_enum : Outport
  wires:
  UnitConverter/1 -> VHAL_HeadLampSW_enum/1
  HeadLampSW/1 -> UnitConverter/1

== system halin/HAL_IN/CAN2/IVI2/HoodLatchSW ==
  Hood_Latch_SW : Inport
  UnitConverter : DataTypeConversion  OutDataTypeStr=uint8
  VHAL_HoodLatchSW_enum : Outport
  wires:
  UnitConverter/1 -> VHAL_HoodLatchSW_enum/1
  Hood_Latch_SW/1 -> UnitConverter/1

== system halin/HAL_IN/CAN2/IVI2/IVIAirIntZ3Cmd ==
  IVI_AirIntZ3_Cmd : Inport
  UnitConverter : DataTypeConversion  OutDataTypeStr=uint8
  VHAL_IVIAirIntZ3Cmd_enum : Outport
  wires:
  UnitConverter/1 -> VHAL_IVIAirIntZ3Cmd_enum/1
  IVI_AirIntZ3_Cmd/1 -> UnitConverter/1

== system halin/HAL_IN/CAN2/IVI2/IVIChargePortSWSta ==
  IVI_ChargePortSW_Sta : Inport
  UnitConverter : DataTypeConversion  OutDataTypeStr=uint8
  VHAL_IVIChargePortSWSta_flg : Outport
  wires:
  UnitConverter/1 -> VHAL_IVIChargePortSWSta_flg/1
  IVI_ChargePortSW_Sta/1 -> UnitConverter/1

== system halin/HAL_IN/CAN2/IVI2/IVICreepSWReq ==
  IVI_CreepSW_Req : Inport
  UnitConverter : DataTypeConversion  OutDataTypeStr=uint8
  VHAL_IVICreepSWReq_flg : Outport
  wires:
  UnitConverter/1 -> VHAL_IVICreepSWReq_flg/1
  IVI_CreepSW_Req/1 -> UnitConverter/1

== system halin/HAL_IN/CAN2/IVI2/IVIDSEATFroEdgeHeightCmd ==
  IVI_DSEAT_FroEdge_Height_Cmd : Inport
  UnitConverter : DataTypeConversion  OutDataTypeStr=uint8
  VHAL_IVIDSEATFroEdgeHeightCmd_enum : Outport
  wires:
  UnitConverter/1 -> VHAL_IVIDSEATFroEdgeHeightCmd_enum/1
  IVI_DSEAT_FroEdge_Height_Cmd/1 -> UnitConverter/1

== system halin/HAL_IN/CAN2/IVI2/IVIDSEATHeaterCmd ==
  IVI_DSEATHeater_Cmd : Inport
  UnitConverter : DataTypeConversion  OutDataTypeStr=uint8
  VHAL_IVIDSEATHeaterCmd_enum : Outport
  wires:
  UnitConverter/1 -> VHAL_IVIDSEATHeaterCmd_enum/1
  IVI_DSEATHeater_Cmd/1 -> UnitConverter/1

== system halin/HAL_IN/CAN2/IVI2/IVIDSEATHeightCmd ==
  IVI_DSEAT_Height_Cmd : Inport
  UnitConverter : DataTypeConversion  OutDataTypeStr=uint8
  VHAL_IVIDSEATHeightCmd_enum : Outport
  wires:
  UnitConverter/1 -> VHAL_IVIDSEATHeightCmd_enum/1
  IVI_DSEAT_Height_Cmd/1 -> UnitConverter/1

== system halin/HAL_IN/CAN2/IVI2/IVIDSEATMemory1Sta ==
  IVI_DSEAT_Memory1_Sta : Inport
  UnitConverter : DataTypeConversion  OutDataTypeStr=uint8
  VHAL_IVIDSEATMemory1Sta_flg : Outport
  wires:
  UnitConverter/1 -> VHAL_IVIDSEATMemory1Sta_flg/1
  IVI_DSEAT_Memory1_Sta/1 -> UnitConverter/1

== system halin/HAL_IN/CAN2/IVI2/IVIDSEATMemory2Sta ==
  IVI_DSEAT_Memory2_Sta : Inport
  UnitConverter : DataTypeConversion  OutDataTypeStr=uint8
  VHAL_IVIDSEATMemory2Sta_flg : Outport
  wires:
  UnitConverter/1 -> VHAL_IVIDSEATMemory2Sta_flg/1
  IVI_DSEAT_Memory2_Sta/1 -> UnitConverter/1

== system halin/HAL_IN/CAN2/IVI2/IVIDSEATMemoryOPTCLSSta ==
  IVI_DSEAT_Memory_OPTCLS_Sta : Inport
  UnitConverter : DataTypeConversion  OutDataTypeStr=uint8
  VHAL_IVIDSEATMemoryOPTCLSSta_flg : Outport
  wires:
  UnitConverter/1 -> VHAL_IVIDSEATMemoryOPTCLSSta_flg/1
  IVI_DSEAT_Memory_OPTCLS_Sta/1 -> UnitConverter/1

== system halin/HAL_IN/CAN2/IVI2/IVIDSEATReclineCmd ==
  IVI_DSEAT_Recline_Cmd : Inport
  UnitConverter : DataTypeConversion  OutDataTypeStr=uint8
  VHAL_IVIDSEATReclineCmd_enum : Outport
  wires:
  UnitConverter/1 -> VHAL_IVIDSEATReclineCmd_enum/1
  IVI_DSEAT_Recline_Cmd/1 -> UnitConverter/1

== system halin/HAL_IN/CAN2/IVI2/IVIDSEATSlideCmd ==
  IVI_DSEAT_Slide_Cmd : Inport
  UnitConverter : DataTypeConversion  OutDataTypeStr=uint8
  VHAL_IVIDSEATSlideCmd_enum : Outport
  wires:
  UnitConverter/1 -> VHAL_IVIDSEATSlideCmd_enum/1
  IVI_DSEAT_Slide_Cmd/1 -> UnitConverter/1

== system halin/HAL_IN/CAN2/IVI2/IVIISAOffsetSpd ==
  IVI_ISA_OffsetSpd : Inport
  UnitConverter : DataTypeConversion  OutDataTypeStr=uint8
  VHAL_IVIISAOffsetSpd_enum : Outport
  wires:
  UnitConverter/1 -> VHAL_IVIISAOffsetSpd_enum/1
  IVI_ISA_OffsetSpd/1 -> UnitConverter/1

== system halin/HAL_IN/CAN2/IVI2/IVINightModeSta ==
  IVI_Night_Mode_Sta : Inport
  UnitConverter : DataTypeConversion  OutDataTypeStr=uint8
  VHAL_IVINightModeSta_flg : Outport
  wires:
  UnitConverter/1 -> VHAL_IVINightModeSta_flg/1
  IVI_Night_Mode_Sta/1 -> UnitConverter/1

== system halin/HAL_IN/CAN2/IVI2/IVIPSEATHeaterCmd ==
  IVI_PSEATHeater_Cmd : Inport
  UnitConverter : DataTypeConversion  OutDataTypeStr=uint8
  VHAL_IVIPSEATHeaterCmd_enum : Outport
  wires:
  UnitConverter/1 -> VHAL_IVIPSEATHeaterCmd_enum/1
  IVI_PSEATHeater_Cmd/1 -> UnitConverter/1

== system halin/HAL_IN/CAN2/IVI2/IVIPSEATReclineCmd ==
  IVI_PSEAT_Recline_Cmd : Inport
  UnitConverter : DataTypeConversion  OutDataTypeStr=uint8
  VHAL_IVIPSEATReclineCmd_enum : Outport
  wires:
  UnitConverter/1 -> VHAL_IVIPSEATReclineCmd_enum/1
  IVI_PSEAT_Recline_Cmd/1 -> UnitConverter/1

== system halin/HAL_IN/CAN2/IVI2/IVIPSEATSlideCmd ==
  IVI_PSEAT_Slide_Cmd : Inport
  UnitConverter : DataTypeConversion  OutDataTypeStr=uint8
  VHAL_IVIPSEATSlideCmd_enum : Outport
  wires:
  UnitConverter/1 -> VHAL_IVIPSEATSlideCmd_enum/1
  IVI_PSEAT_Slide_Cmd/1 -> UnitConverter/1

== system halin/HAL_IN/CAN2/IVI2/IVIPTGModeSW ==
  IVI_PTG_Mode_SW : Inport
  UnitConverter : DataTypeConversion  OutDataTypeStr=uint8
  VHAL_IVIPTGModeSW_enum : Outport
  wires:
  UnitConverter/1 -> VHAL_IVIPTGModeSW_enum/1
  IVI_PTG_Mode_SW/1 -> UnitConverter/1

== system halin/HAL_IN/CAN2/IVI2/IVIPTGOpenHeight ==
  IVI_PTG_Open_Height : Inport
  UnitConverter : DataTypeConversion  OutDataTypeStr=uint8
  VHAL_IVIPTGOpenHeight_enum : Outport
  wires:
  UnitConverter/1 -> VHAL_IVIPTGOpenHeight_enum/1
  IVI_PTG_Open_Height/1 -> UnitConverter/1

== system halin/HAL_IN/CAN2/IVI2/IVIPTGStaSW ==
  IVI_PTG_Sta_SW : Inport
  UnitConverter : DataTypeConversion  OutDataTypeStr=uint8
  VHAL_IVIPTGStaSW_enum : Outport
  wires:
  UnitConverter/1 -> VHAL_IVIPTGStaSW_enum/1
  IVI_PTG_Sta_SW/1 -> UnitConverter/1

== system halin/HAL_IN/CAN2/IVI2/IVIPTGUSStaSW ==
  IVI_PTG_USSta_SW : Inport
  UnitConverter : DataTypeConversion  OutDataTypeStr=uint8
  VHAL_IVIPTGUSStaSW_flg : Outport
  wires:
  UnitConverter/1 -> VHAL_IVIPTGUSStaSW_flg/1
  IVI_PTG_USSta_SW/1 -> UnitConverter/1

== system halin/HAL_IN/CAN2/IVI2/IVIPWModeReq ==
  IVI_PW_Mode_Req : Inport
  UnitConverter : DataTypeConversion  OutDataTypeStr=uint8
  VHAL_IVIPWModeReq_enum : Outport
  wires:
  UnitConverter/1 -> VHAL_IVIPWModeReq_enum/1
  IVI_PW_Mode_Req/1 -> UnitConverter/1

== system halin/HAL_IN/CAN2/IVI2/IVIPwrLockSW ==
  IVI_PwrLockSW : Inport
  UnitConverter : DataTypeConversion  OutDataTypeStr=uint8
  VHAL_IVIPwrLockSW_enum : Outport
  wires:
  UnitConverter/1 -> VHAL_IVIPwrLockSW_enum/1
  IVI_PwrLockSW/1 -> UnitConverter/1

== system halin/HAL_IN/CAN2/IVI2/IVIPwroffreq ==
  IVI_Pwroff_req : Inport
  UnitConverter : DataTypeConversion  OutDataTypeStr=uint8
  VHAL_IVIPwroffreq_flg : Outport
  wires:
  UnitConverter/1 -> VHAL_IVIPwroffreq_flg/1
  IVI_Pwroff_req/1 -> UnitConverter/1

== system halin/HAL_IN/CAN2/IVI2/IVIRRDefReq ==
  IVI_RR_Def_Req : Inport
  UnitConverter : DataTypeConversion  OutDataTypeStr=uint8
  VHAL_IVIRRDefReq_flg : Outport
  wires:
  UnitConverter/1 -> VHAL_IVIRRDefReq_flg/1
  IVI_RR_Def_Req/1 -> UnitConverter/1

== system halin/HAL_IN/CAN2/IVI2/IVIReqV2L ==
  IVI_Req_V2L : Inport
  UnitConverter : DataTypeConversion  OutDataTypeStr=uint8
  VHAL_IVIReqV2L_enum : Outport
  wires:
  UnitConverter/1 -> VHAL_IVIReqV2L_enum/1
  IVI_Req_V2L/1 -> UnitConverter/1

== system halin/HAL_IN/CAN2/IVI2/IVIScreen ==
  IVI_Screen : Inport
  UnitConverter : DataTypeConversion  OutDataTypeStr=uint8
  VHAL_IVIScreen_enum : Outport
  wires:
  UnitConverter/1 -> VHAL_IVIScreen_enum/1
  IVI_Screen/1 -> UnitConverter/1

== system halin/HAL_IN/CAN2/IVI2/IVIStartChgreq ==
  IVI_Start_Chg_req : Inport
  UnitConverter : DataTypeConversion  OutDataTypeStr=uint8
  VHAL_IVIStartChgreq_flg : Outport
  wires:
  UnitConverter/1 -> VHAL_IVIStartChgreq_flg/1
  IVI_Start_Chg_req/1 -> UnitConverter/1

== system halin/HAL_IN/CAN2/IVI2/IVIStatus ==
  IVI_Status : Inport
  UnitConverter : DataTypeConversion  OutDataTypeStr=uint8
  VHAL_IVIStatus_flg : Outport
  wires:
  UnitConverter/1 -> VHAL_IVIStatus_flg/1
  IVI_Status/1 -> UnitConverter/1

== system halin/HAL_IN/CAN2/IVI2/IVIStopChgreq ==
  IVI_Stop_Chg_req : Inport
  UnitConverter : DataTypeConversion  OutDataTypeStr=uint8
  VHAL_IVIStopChgreq_flg : Outport
  wires:
  UnitConverter/1 -> VHAL_IVIStopChgreq_flg/1
  IVI_Stop_Chg_req/1 -> UnitConverter/1

== system halin/HAL_IN/CAN2/IVI2/IVITrailerCheckReqSta ==
  IVI_TrailerCheckReq_Sta : Inport
  UnitConverter : DataTypeConversion  OutDataTypeStr=uint8
  VHAL_IVITrailerCheckReqSta_flg : Outport
  wires:
  UnitConverter/1 -> VHAL_IVITrailerCheckReqSta_flg/1
  IVI_TrailerCheckReq_Sta/1 -> UnitConverter/1

== system halin/HAL_IN/CAN2/IVI2/IVITrailerModeSWSta ==
  IVI_TrailerModeSW_Sta : Inport
  UnitConverter : DataTypeConversion  OutDataTypeStr=uint8
  VHAL_IVITrailerModeSWSta_flg : Outport
  wires:
  UnitConverter/1 -> VHAL_IVITrailerModeSWSta_flg/1
  IVI_TrailerModeSW_Sta/1 -> UnitConverter/1

== system halin/HAL_IN/CAN2/IVI2/IVITriggerreq ==
  IVI_Trigger_req : Inport
  UnitConverter : DataTypeConversion  OutDataTypeStr=uint8
  VHAL_IVITriggerreq_flg : Outport
  wires:
  UnitConverter/1 -> VHAL_IVITriggerreq_flg/1
  IVI_Trigger_req/1 -> UnitConverter/1

== system halin/HAL_IN/CAN2/IVI2/IVIUnlockChgreq ==
  IVI_Unlock_Chg_req : Inport
  UnitConverter : DataTypeConversion  OutDataTypeStr=uint8
  VHAL_IVIUnlockChgreq_flg : Outport
  wires:
  UnitConverter/1 -> VHAL_IVIUnlockChgreq_flg/1
  IVI_Unlock_Chg_req/1 -> UnitConverter/1

== system halin/HAL_IN/CAN2/IVI2/IVIWIMAINSW ==
  IVI_WI_MAIN_SW : Inport
  UnitConverter : DataTypeConversion  OutDataTypeStr=uint8
  VHAL_IVIWIMAINSW_flg : Outport
  wires:
  UnitConverter/1 -> VHAL_IVIWIMAINSW_flg/1
  IVI_WI_MAIN_SW/1 -> UnitConverter/1

== system halin/HAL_IN/CAN2/IVI2/LDrvControlCommand ==
  L_Drv_ControlCommand : Inport
  UnitConverter : DataTypeConversion  OutDataTypeStr=uint8
  VHAL_LDrvControlCommand_pct : Outport
  wires:
  UnitConverter/1 -> VHAL_LDrvControlCommand_pct/1
  L_Drv_ControlCommand/1 -> UnitConverter/1

== system halin/HAL_IN/CAN2/IVI2/LPasControlCommand ==
  L_Pas_ControlCommand : Inport
  UnitConverter : DataTypeConversion  OutDataTypeStr=uint8
  VHAL_LPasControlCommand_pct : Outport
  wires:
  UnitConverter/1 -> VHAL_LPasControlCommand_pct/1
  L_Pas_ControlCommand/1 -> UnitConverter/1

== system halin/HAL_IN/CAN2/IVI2/LRLDControlCommand ==
  L_RLD_ControlCommand : Inport
  UnitConverter : DataTypeConversion  OutDataTypeStr=uint8
  VHAL_LRLDControlCommand_pct : Outport
  wires:
  UnitConverter/1 -> VHAL_LRLDControlCommand_pct/1
  L_RLD_ControlCommand/1 -> UnitConverter/1

== system halin/HAL_IN/CAN2/IVI2/LRRDControlCommand ==
  L_RRD_ControlCommand : Inport
  UnitConverter : DataTypeConversion  OutDataTypeStr=uint8
  VHAL_LRRDControlCommand_pct : Outport
  wires:
  UnitConverter/1 -> VHAL_LRRDControlCommand_pct/1
  L_RRD_ControlCommand/1 -> UnitConverter/1

== system halin/HAL_IN/CAN2/IVI2/LightShowStartReq ==
  Light_ShowStart_Req : Inport
  UnitConverter : DataTypeConversion  OutDataTypeStr=uint8
  VHAL_LightShowStartReq_flg : Outport
  wires:
  UnitConverter/1 -> VHAL_LightShowStartReq_flg/1
  Light_ShowStart_Req/1 -> UnitConverter/1

== system halin/HAL_IN/CAN2/IVI2/LightShowStopReq ==
  Light_ShowStop_Req : Inport
  UnitConverter : DataTypeConversion  OutDataTypeStr=uint8
  VHAL_LightShowStopReq_flg : Outport
  wires:
  UnitConverter/1 -> VHAL_LightShowStopReq_flg/1
  Light_ShowStop_Req/1 -> UnitConverter/1

== system halin/HAL_IN/CAN2/IVI2/MFRDNBrightReq ==
  MFRD_N_Bright_Req : Inport
  UnitConverter : DataTypeConversion  OutDataTypeStr=uint8
  VHAL_MFRDNBrightReq_pct : Outport
  wires:
  UnitConverter/1 -> VHAL_MFRDNBrightReq_pct/1
  MFRD_N_Bright_Req/1 -> UnitConverter/1

== system halin/HAL_IN/CAN2/IVI2/OFFACMODE ==
  OFF_AC_MODE : Inport
  UnitConverter : DataTypeConversion  OutDataTypeStr=uint8
  VHAL_OFFACMODE_enum : Outport
  wires:
  UnitConverter/1 -> VHAL_OFFACMODE_enum/1
  OFF_AC_MODE/1 -> UnitConverter/1

== system halin/HAL_IN/CAN2/IVI2/PSEATventreq ==
  PSEAT_vent_req : Inport
  UnitConverter : DataTypeConversion  OutDataTypeStr=uint8
  VHAL_PSEATventreq_enum : Outport
  wires:
  UnitConverter/1 -> VHAL_PSEATventreq_enum/1
  PSEAT_vent_req/1 -> UnitConverter/1

== system halin/HAL_IN/CAN2/IVI2/PerdV2L ==
  Perd_V2L : Inport
  UnitConverter : DataTypeConversion  OutDataTypeStr=uint8
  VHAL_PerdV2L_enum : Outport
  wires:
  UnitConverter/1 -> VHAL_PerdV2L_enum/1
  Perd_V2L/1 -> UnitConverter/1

== system halin/HAL_IN/CAN2/IVI2/RFogLampSW ==
  RFogLampSW : Inport
  UnitConverter : DataTypeConversion  OutDataTypeStr=uint8
  VHAL_RFogLampSW_flg : Outport
  wires:
  UnitConverter/1 -> VHAL_RFogLampSW_flg/1
  RFogLampSW/1 -> UnitConverter/1

== system halin/HAL_IN/CAN2/IVI2/RollModeSWCmd ==
  Roll_Mode_SW_Cmd : Inport
  UnitConverter : DataTypeConversion  OutDataTypeStr=uint8
  VHAL_RollModeSWCmd_enum : Outport
  wires:
  UnitConverter/1 -> VHAL_RollModeSWCmd_enum/1
  Roll_Mode_SW_Cmd/1 -> UnitConverter/1

== system halin/HAL_IN/CAN2/IVI2/RoomLampMode ==
  RoomLampMode : Inport
  UnitConverter : DataTypeConversion  OutDataTypeStr=uint8
  VHAL_RoomLampMode_flg : Outport
  wires:
  UnitConverter/1 -> VHAL_RoomLampMode_flg/1
  RoomLampMode/1 -> UnitConverter/1

== system halin/HAL_IN/CAN2/IVI2/SOCADJBUTT ==
  SOC_ADJ_BUTT : Inport
  UnitConverter : DataTypeConversion  OutDataTypeStr=uint8
  VHAL_SOCADJBUTT_flg : Outport
  wires:
  UnitConverter/1 -> VHAL_SOCADJBUTT_flg/1
  SOC_ADJ_BUTT/1 -> UnitConverter/1

== system halin/HAL_IN/CAN2/IVI2/SOCLimitSet ==
  SOC_Limit_Set : Inport
  UnitConverter : DataTypeConversion  OutDataTypeStr=uint8
  convert_in : FVT_lib/hal/convert_in  gain=2  offset=50
  VHAL_SOCLimitSet_pct : Outport
  wires:
  convert_in/1 -> VHAL_SOCLimitSet_pct/1
  UnitConverter/1 -> convert_in/1
  SOC_Limit_Set/1 -> UnitConverter/1

== system halin/HAL_IN/CAN2/IVI2/SOCV2LLimit ==
  SOC_V2LLimit : Inport
  UnitConverter : DataTypeConversion  OutDataTypeStr=uint8
  convert_in : FVT_lib/hal/convert_in  gain=5  offset=20
  VHAL_SOCV2LLimit_pct : Outport
  wires:
  convert_in/1 -> VHAL_SOCV2LLimit_pct/1
  UnitConverter/1 -> convert_in/1
  SOC_V2LLimit/1 -> UnitConverter/1

== system halin/HAL_IN/CAN2/IVI2/SchedChgStart ==
  Sched_Chg_Start : Inport
  UnitConverter : DataTypeConversion  OutDataTypeStr=uint8
  VHAL_SchedChgStart_flg : Outport
  wires:
  UnitConverter/1 -> VHAL_SchedChgStart_flg/1
  Sched_Chg_Start/1 -> UnitConverter/1

== system halin/HAL_IN/CAN2/IVI2/SchedChgStop ==
  Sched_Chg_Stop : Inport
  UnitConverter : DataTypeConversion  OutDataTypeStr=uint8
  VHAL_SchedChgStop_flg : Outport
  wires:
  UnitConverter/1 -> VHAL_SchedChgStop_flg/1
  Sched_Chg_Stop/1 -> UnitConverter/1

== system halin/HAL_IN/CAN2/IVI2/SchedChgbutt ==
  Sched_Chg_butt : Inport
  UnitConverter : DataTypeConversion  OutDataTypeStr=uint8
  VHAL_SchedChgbutt_flg : Outport
  wires:
  UnitConverter/1 -> VHAL_SchedChgbutt_flg/1
  Sched_Chg_butt/1 -> UnitConverter/1

== system halin/HAL_IN/CAN2/IVI2/SchedChglimit ==
  Sched_Chg_limit : Inport
  UnitConverter : DataTypeConversion  OutDataTypeStr=uint8
  convert_in : FVT_lib/hal/convert_in  gain=2  offset=50
  VHAL_SchedChglimit_pct : Outport
  wires:
  convert_in/1 -> VHAL_SchedChglimit_pct/1
  UnitConverter/1 -> convert_in/1
  Sched_Chg_limit/1 -> UnitConverter/1

== system halin/HAL_IN/CAN2/IVI2/SchedChgwake ==
  Sched_Chg_wake : Inport
  UnitConverter : DataTypeConversion  OutDataTypeStr=uint8
  VHAL_SchedChgwake_flg : Outport
  wires:
  UnitConverter/1 -> VHAL_SchedChgwake_flg/1
  Sched_Chg_wake/1 -> UnitConverter/1

== system halin/HAL_IN/CAN2/IVI2/SenstivityPosition ==
  SenstivityPosition : Inport
  UnitConverter : DataTypeConversion  OutDataTypeStr=uint8
  VHAL_SenstivityPosition_enum : Outport
  wires:
  UnitConverter/1 -> VHAL_SenstivityPosition_enum/1
  SenstivityPosition/1 -> UnitConverter/1

== system halin/HAL_IN/CAN2/IVI2/SetUnlockSingle ==
  SetUnlockSingle : Inport
  UnitConverter : DataTypeConversion  OutDataTypeStr=uint8
  VHAL_SetUnlockSingle_flg : Outport
  wires:
  UnitConverter/1 -> VHAL_SetUnlockSingle_flg/1
  SetUnlockSingle/1 -> UnitConverter/1

== system halin/HAL_IN/CAN2/IVI2/TCSSWCmd ==
  TCS_SW_Cmd : Inport
  UnitConverter : DataTypeConversion  OutDataTypeStr=uint8
  VHAL_TCSSWCmd_enum : Outport
  wires:
  UnitConverter/1 -> VHAL_TCSSWCmd_enum/1
  TCS_SW_Cmd/1 -> UnitConverter/1

== system halin/HAL_IN/CAN2/IVI2/TPMSCaliButt ==
  TPMS_Cali_Butt : Inport
  UnitConverter : DataTypeConversion  OutDataTypeStr=uint8
  VHAL_TPMSCaliButt_flg : Outport
  wires:
  UnitConverter/1 -> VHAL_TPMSCaliButt_flg/1
  TPMS_Cali_Butt/1 -> UnitConverter/1

== system halin/HAL_IN/CAN2/IVI2/TPMSResButt ==
  TPMS_Res_Butt : Inport
  UnitConverter : DataTypeConversion  OutDataTypeStr=uint8
  VHAL_TPMSResButt_flg : Outport
  wires:
  UnitConverter/1 -> VHAL_TPMSResButt_flg/1
  TPMS_Res_Butt/1 -> UnitConverter/1

== system halin/HAL_IN/CAN2/IVI2/TurnSwTimeSet ==
  TurnSwTimeSet : Inport
  UnitConverter : DataTypeConversion  OutDataTypeStr=uint8
  VHAL_TurnSwTimeSet_enum : Outport
  wires:
  UnitConverter/1 -> VHAL_TurnSwTimeSet_enum/1
  TurnSwTimeSet/1 -> UnitConverter/1

== system halin/HAL_IN/CAN2/IVI2/WalkawayLockSW ==
  Walkaway_Lock_SW : Inport
  UnitConverter : DataTypeConversion  OutDataTypeStr=uint8
  VHAL_WalkawayLockSW_flg : Outport
  wires:
  UnitConverter/1 -> VHAL_WalkawayLockSW_flg/1
  Walkaway_Lock_SW/1 -> UnitConverter/1

== system halin/HAL_IN/CAN2/IVI2/WlcmLightMode ==
  WlcmLight_Mode : Inport
  UnitConverter : DataTypeConversion  OutDataTypeStr=uint8
  VHAL_WlcmLightMode_enum : Outport
  wires:
  UnitConverter/1 -> VHAL_WlcmLightMode_enum/1
  WlcmLight_Mode/1 -> UnitConverter/1

== system halin/HAL_IN/CAN2/IVI2/sigAirIntenZon1Req ==
  sigAirIntenZon1Req : Inport
  UnitConverter : DataTypeConversion  OutDataTypeStr=uint8
  VHAL_sigAirIntenZon1Req_enum : Outport
  wires:
  UnitConverter/1 -> VHAL_sigAirIntenZon1Req_enum/1
  sigAirIntenZon1Req/1 -> UnitConverter/1

== system halin/HAL_IN/CAN2/IVI2/sigDfrstReq ==
  sigDfrstReq : Inport
  UnitConverter : DataTypeConversion  OutDataTypeStr=uint8
  VHAL_sigDfrstReq_flg : Outport
  wires:
  UnitConverter/1 -> VHAL_sigDfrstReq_flg/1
  sigDfrstReq/1 -> UnitConverter/1

== system halin/HAL_IN/CAN2/IVI2/sigFaceReq ==
  sigFaceReq : Inport
  UnitConverter : DataTypeConversion  OutDataTypeStr=uint8
  VHAL_sigFaceReq_flg : Outport
  wires:
  UnitConverter/1 -> VHAL_sigFaceReq_flg/1
  sigFaceReq/1 -> UnitConverter/1

== system halin/HAL_IN/CAN2/IVI2/sigFootReq ==
  sigFootReq : Inport
  UnitConverter : DataTypeConversion  OutDataTypeStr=uint8
  VHAL_sigFootReq_flg : Outport
  wires:
  UnitConverter/1 -> VHAL_sigFootReq_flg/1
  sigFootReq/1 -> UnitConverter/1

== system halin/HAL_IN/CAN2/IVI2/sigRecircReq ==
  sigRecircReq : Inport
  UnitConverter : DataTypeConversion  OutDataTypeStr=uint8
  VHAL_sigRecircReq_flg : Outport
  wires:
  UnitConverter/1 -> VHAL_sigRecircReq_flg/1
  sigRecircReq/1 -> UnitConverter/1

== system halin/HAL_IN/CAN2/IVI2/sigSetTempZon1Req ==
  sigSetTempZon1Req : Inport
  UnitConverter : DataTypeConversion  OutDataTypeStr=uint8
  convert_in : FVT_lib/hal/convert_in  gain=0.5  offset=17
  VHAL_sigSetTempZon1Req_C : Outport
  wires:
  convert_in/1 -> VHAL_sigSetTempZon1Req_C/1
  UnitConverter/1 -> convert_in/1
  sigSetTempZon1Req/1 -> UnitConverter/1

== system halin/HAL_IN/CAN2/IVI2/sigSetTempZon2Req ==
  sigSetTempZon2Req : Inport
  UnitConverter : DataTypeConversion  OutDataTypeStr=uint8
  convert_in : FVT_lib/hal/convert_in  gain=0.5  offset=17
  VHAL_sigSetTempZon2Req_C : Outport
  wires:
  convert_in/1 -> VHAL_sigSetTempZon2Req_C/1
  UnitConverter/1 -> convert_in/1
  sigSetTempZon2Req/1 -> UnitConverter/1
